simulink model "PID_Pendule"  (R2025a)
settings: Solver=VariableStepAuto  StartTime=0.0  StopTime=10  RelTol=1e-3
values from neighbouring files (symbols this model uses):
  A = [0 1 ... (first row only)    [pendule.m]    (also in pendule_obs.m)
  B = [0 ... (first row only)    [pendule.m]    (also in pendule_obs.m)
  C = [1 0]    [pendule.m]    (also in pendule_obs.m)
  D = 0    [pendule_obs.m]
  K = place(A, B, [-1 -1.5])    [pendule_obs.m]
  theta_r = pi/3    (= 1.0471975512)    [pendule.m]    (also in pendule_obs.m)
  X0 = [theta_0; omega_0]    [pendule_obs.m]
settings Model: Creator=vikfo  LastModifiedBy=vikfo

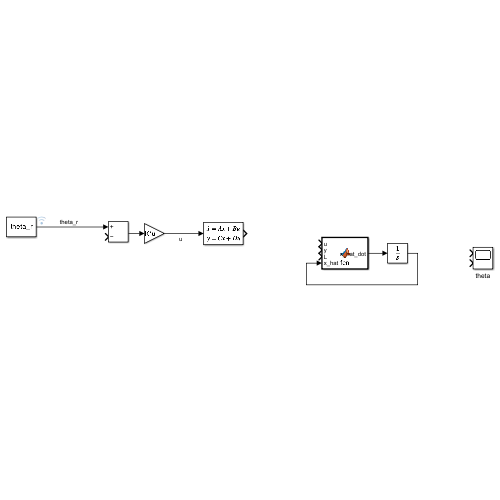
[thumbnail: Simulink's stored preview of the top-level diagram]
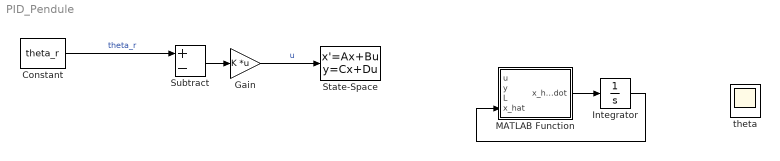
== system PID_Pendule ==
  Constant : Constant  Value=theta_r
  Gain : Gain  Gain=K  Multiplication=Matrix(K*u)
  Integrator : Integrator
  MATLAB Function : MATLAB Function  TreatAsAtomicUnit=on
  State-Space : StateSpace  A=A  B=B  C=C  D=D  InitialCondition=X0
  Subtract : Sum  Inputs=+-
  theta : Scope  NumInputPorts=2
      settings: ActiveDisplayYMinimum=0.42158126344051738  ActiveDisplayYMaximum=1.4417563850183324
  wires:
  Subtract/1 -> Gain/1
  Gain/1 -> State-Space/1  "u"
  Constant/1 -> Subtract/1  "theta_r"
  MATLAB Function/1(x_hat_dot) -> Integrator/1
  Integrator/1 -> MATLAB Function/4(x_hat)

== matlab function PID_Pendule/MATLAB Function ==
  data: u input; x_hat_dot output; y input; L input; x_hat input
function x_hat_dot = fcn(u, y, L,x_hat)



y = u;
